simulink model "GCAWS"  (R2022a)
settings: Solver=FixedStepDiscrete  StartTime=0.0  StopTime=1  FixedStep=0.04  RelTol=1e-3
PreLoadFcn:
  | % Add Module Path
  | listing = dir;
  | if (contains([listing .name], 'TCAF')) && (contains([listing .name], 'MAP'))
  |     addpath('./TCAF', './MAP');
  |     addpath( genpath('./MAP') );
  | elseif (contains([listing .name], 'GCAWS.slx'))
  |     addpath('../TCAF', '../MAP');
  |     addpath( genpath('../MAP') );
  | else
  | end
  | 
  | % Add DataBus Path
  | load('BusStructureGCAWS.mat');
  | load('BusStructureWTPG.mat');
  | load('TRN\BusStructureTRN.mat');
InitFcn:
  | % Add Module Path
  | listing = dir;
  | if (contains([listing .name], 'TCAF')) && (contains([listing .name], 'MAP'))
  |     addpath('./TCAF', './MAP');
  |     addpath( genpath('./MAP') );
  | elseif (contains([listing .name], 'GCAWS.slx'))
  |     addpath('../TCAF', '../MAP');
  |     addpath( genpath('../MAP') );
  | else
  | end
  | 
  | % Add DataBus Path
  | load('BusStructureGCAWS.mat');
  | load('BusStructureWTPG.mat');
  | load('TRN\BusStructureTRN.mat');
StartFcn:
  | % Add Module Path
  | listing = dir;
  | if (contains([listing .name], 'TCAF')) && (contains([listing .name], 'MAP'))
  |     addpath('./TCAF', './MAP');
  |     addpath( genpath('./MAP') );
  | elseif (contains([listing .name], 'GCAWS.slx'))
  |     addpath('../TCAF', '../MAP');
  |     addpath( genpath('../MAP') );
  | else
  | end
  | 
  | % Add DataBus Path
  | load('BusStructureGCAWS.mat');
  | load('BusStructureWTPG.mat');
  | load('TRN\BusStructureTRN.mat');
values from neighbouring files (symbols this model uses):
  isFeasible = logsout{idx_WTPGDatapump}.Values.isFeasible.Data(ii,:)    [WTPG_SIM_AFTERPLOT.m]
undefined symbols (not defined in the file or in its folder): accNED, C_b_n, collisionWarning, collisionWarningValid, gOnsetRateWrap, lla, maxFlightPathAngleWrap, offObstructionMap, offTerrainMap, params, paramSelectedValid, pullUpGWrap, reactionTimeWrap, rollRateWrap, selectedWrap, statusCode, timeToGoToPullUp, velNED
libraries: hdlsllib x15, simulink x2
(part 2 of 2)

== matlab function GCAWS/ImplementGCAWS/CheckCollision/FindPullUpTimeLeft/BisectPullUpTimeBackup ==
  data: collisionFlag input; collisionIndex input; pullUpT output; predTraj input; hulledProfile input
function pullUpT = BisectPullUpTime(collisionFlag, collisionIndex, predTraj, hulledProfile)
%BisectPullUpTime
% == Output =======
% pullUpT : Time to pull-up time left [sec]

% Initailize output
pullUpT = single(10);
pullUpTD = 0;
terrHR = 0;
terrHL = 0;
terrTest = 0;

DELTA_T = 0.5;

% % If no collision found in the projected trajectory, return
% if collisionFlag(1) == 10
%     pullUpT = single(10);
%     return
% end

% If no collision found in pull-up trajectories, return
if (collisionFlag(2) == 65535) || (collisionFlag(1) == 65535) || (collisionIndex(2) == 65535)
    pullUpT = single(10);
    return
elseif ( (collisionIndex(2)-1) == 0 )
    % Collision now
    pullUpT = single(0);
    return;
else
    % Initialize TTGTPU
    pullUpTD = double( collisionIndex(2)-1 ) * DELTA_T;
    % Terrain Height at collision detected point
    terrHR = double( hulledProfile(collisionIndex(2)) );

    stateL = [ predTraj(collisionIndex(2)-1, collisionFlag(2), 1), ...
        predTraj(collisionIndex(2)-1, collisionFlag(2), 2), ...
        predTraj(collisionIndex(2)-1, collisionFlag(2), 3), ...
        pullUpTD-DELTA_T ];
    stateR = [ predTraj(collisionIndex(2), collisionFlag(2), 1), ...
        predTraj(collisionIndex(2), collisionFlag(2), 2), ...
        predTraj(collisionIndex(2), collisionFlag(2), 3), ...
        pullUpTD ];
    % Terrain height just before collision detected point
    terrHL = double( hulledProfile(collisionIndex(2)-1) );

    for bb = 0:12
        % Test terrain height

        terrTest = terrHL * ( (pullUpTD - (stateL(4) + stateR(4))/2 ) / DELTA_T) + ...
            terrHR * ( 1 - (pullUpTD - (stateL(4) + stateR(4))/2 ) / DELTA_T);

%         if ( abs(terrTest-((stateL(3) + stateR(3))/2)) < 0.01 )
%             break;
%         end

        if ( terrTest > ((stateL(3) + stateR(3))/2) )
            stateR(1) = (stateL(1) + stateR(1)) /2;
            stateR(2) = (stateL(2) + stateR(2)) /2;
            stateR(3) = (stateL(3) + stateR(3)) /2;
            stateR(4) = (stateL(4) + stateR(4)) /2;

        else
            stateL(1) = (stateL(1) + stateR(1)) /2;
            stateL(2) = (stateL(2) + stateR(2)) /2;
            stateL(3) = (stateL(3) + stateR(3)) /2;
            stateL(4) = (stateL(4) + stateR(4)) /2;

        end
    end

end

pullUpT = single( (stateL(4) + stateR(4))/2 );

end

== matlab function GCAWS/ImplementGCAWS/PredictTrajectory/GetProjectTrajectory ==
  data: GCAWSParam input; predTraj input; eulerDeg input; velXYZ input; velNED input; accXYZ input; lla input; predTraj output
function predTraj = GetProjectTrajectory(GCAWSParam, predTraj, eulerDeg, velXYZ, velNED, accXYZ, lla)
%GetProjectTrajectory GCAWS 명목 궤적 생성
%
% == Input =========
% GCAWSParam = [reactT; gMax; rollRate; gRate; gammaMax]
% predTraj - size of [41, 12, 3]
% eulerDeg = [roll; pitch; heading] (deg)
% velXYZ = [celX; velY; velZ] (mps)
% velNED = [velN; velE; velD] (mps)
% accXYZ = [accX; accY; accZ] (mps2)
% lla = [latitude_deg; longitude_deg; altitude_msl_m]
% DELTA_T = 0.5
% == Output ========
% predTraj = [41, 12, 3]
% 

% Define Constants
ALONG_TRACK_STEPS = size(predTraj, 1);
DELTA_T = 0.5;

%% Trajectory Prediction

% <1> Non-Pull-Up Scenario
predTraj(:, 1, :) = projectTrajcetory(eulerDeg, velXYZ, velNED, accXYZ, lla, ALONG_TRACK_STEPS, DELTA_T);
end

%% Internal functions
function nominal = projectTrajcetory(eulerDeg, velXYZ, velNED, accXYZ, lla, ALONG_TRACK_STEPS, DELTA_T)
%PROJECTTRAJECTORY
% Nominal Trajcetory 명목 궤적 예측
%       - Assumption 1: current aircraft sate is 100% reliable
%       - Assumption 2: aircraft maneuver is maintained

% Define constants
GRAV_ACC = 9.8;
LIMIT_TAN_ROL = 4;
LIMIT_TURN_RATE = 0.222; % [rad/s]
RAD2DEG = 180/pi;

assert (ALONG_TRACK_STEPS <= 81);

% Input Handling
rol = eulerDeg(1);
pit = eulerDeg(2);
hdg = eulerDeg(3);

velX = velXYZ(1);
velY = velXYZ(2);
velZ = velXYZ(3);

velN = velNED(1);
velE = velNED(2);
velD = velNED(3);

lat = lla(1);
lon = lla(2);
alt = lla(3);

% Flight path angle (deg)
gamma = atan2d(-velD, sqrt(velN^2+velE^2));

% Inertial speed
iSpd = sqrt( velX^2 + velY^2 + velZ^2 );
    
% Saturate inertial speed (since TAS is unavailable, use inertial spd) 
iSpd = saturate(iSpd, 0.1, 500);

% Calculate the length of a degree
[latLength, lonLength] = getLengthOfADegree(lat, alt);

velLat = velN / latLength;
velLon = velE / lonLength;

% Initialize Predicted Trajectory
nominal = zeros(ALONG_TRACK_STEPS, 1, 3);

% Start point
nominal(1, 1, 1) = lat;
nominal(1, 1, 2) = lon;
nominal(1, 1, 3) = alt;

for ii = 2:ALONG_TRACK_STEPS
    
    % [1] Update Attitude
    
    % Saturate tangent of roll (max bank angle = 75.9630 deg)
    tanRol = saturate(tand(rol), -LIMIT_TAN_ROL, LIMIT_TAN_ROL);
    
    % Saturate inertial speed (since TAS is unavailable, use inertial spd) 
    iSpd = saturate(iSpd, 0.1, 500);
    
    % Calculate turn rate [rad/s]
    turnRate = GRAV_ACC * tanRol / iSpd;
    
    % Saturate turn rate 
    turnRate = saturate(turnRate, -LIMIT_TURN_RATE, LIMIT_TURN_RATE);
        
    % Update heading [deg]
    hdg = hdg + turnRate * DELTA_T * RAD2DEG;
        
    % Update Flight Path Angle [deg]
    %        reaction time: 1.5 sec
    %        rate of change: 5 deg/s
    if ii < 4
        gamma = gamma;
    elseif gamma < -(5*DELTA_T)
        gamma = gamma + 5 * DELTA_T;
    elseif gamma < 0.0
        gamma = 0.0;
    else
        gamma = gamma;
    end

    % [2] Update Velocity
    velNTmp = sqrt(velN^2+velE^2+velD^2)*cosd(hdg)*cosd(gamma);
    velE    = sqrt(velN^2+velE^2+velD^2)*sind(hdg)*cosd(gamma);
    velN    = velNTmp;
    velDOld = velD;
    velD    = - sqrt(velN^2+velE^2+velD^2)*sind(gamma);

    % [3] Update Position
    % Rate of change in geodetic coordinates [deg/s]
    [latLength, lonLength] = getLengthOfADegree(nominal(ii, 1, 1), nominal(ii, 1, 3));
    velLatOld = velLat;
    velLonOld = velLon;
    velLat  = velN / latLength;
    velLon  = velE / lonLength;
    
    nominal(ii, 1, 1) = nominal(ii-1, 1, 1) + (velLat + velLatOld)/2 * DELTA_T;
    nominal(ii, 1, 2) = nominal(ii-1, 1, 2) + (velLon + velLonOld)/2 * DELTA_T;
    nominal(ii, 1, 3) = nominal(ii-1, 1, 3) - (velD + velDOld)/2 * DELTA_T;

end

end

function out = saturate(in, minVal, maxVal)
%SATURATE
% Saturates input value to [min, max]
%
% == Inputs =========
% in                - input value
% minVal            - minimum value
% maxVal            - maximum value
% == Outputs ========
% out               - saturated output value
% ===================

out = min(maxVal, max(minVal, in));

end

function [latLength, lonLength] = getLengthOfADegree(lat, h)
%GETLENGTHOFADEGREE
% Calculate the length of one degree of both latitude and longitude
% for a specified latitude and height
%
% == Inputs =========
% lat               - Latitude [deg]
% h                 - Height [m]
% 
% == Outputs ========
% latLength         - Length of 1 deg of latitude on the ref. spheroid [m]
% lonLength         - Length of 1 deg of longitude on the ref. spheroid [m]
% ===================

% WGS84 Parameters
eRadius = 6378137.0;
eEccen = 0.08181919;

% Radius of curvature in prime vertical
nE = eRadius / sqrt( 1 - (eEccen^2*(sind(lat))^2) );
% Meridian Radius of Curavature
mE = eRadius * (1 - eEccen^2) / (1 - eEccen^2*(sind(lat))^2)^(1.5);

lonLength = (nE + h) * cosd(lat) * (pi/180);
latLength = (mE + h) * (pi/180);

end

== matlab function GCAWS/HandleGCAWSInput/ConvertBody2NED ==
  data: eulerDeg input; vecNED output; vecXYZ input; C_b_n output
function [vecNED, C_b_n] = ConvertBody2NED(eulerDeg, vecXYZ)
%CONVERTBODY2NED 동체 좌표계 벡터를 NED 좌표계 벡터로 변환
% Body2NED 변환 행렬 출력

% Initialize
vecNED = zeros(3,1);
C_b_n = zeros(3,3);

% Trigonometirc functions
cRol = cosd(eulerDeg(1));
sRol = sind(eulerDeg(1));
cPit = cosd(eulerDeg(2));
sPit = sind(eulerDeg(2));
cYaw = cosd(eulerDeg(3));
sYaw = sind(eulerDeg(3));

% Transformation matrix
C_b_n   = [ cPit*cYaw, sRol*sPit*cYaw-cRol*sYaw, cRol*sPit*cYaw+sRol*sYaw;...
            cPit*sYaw, sRol*sPit*sYaw+cRol*cYaw, cRol*sPit*sYaw-sRol*cYaw;...
                -sPit,                sRol*cPit,                cRol*cPit];

% Transform
vecNED = C_b_n * vecXYZ;

end

== matlab function GCAWS/ImplementGCAWS/CheckCollision/FindCollisionFlag ==
  data: collision input; collisionFlag output; collisionIndex output
function [collisionFlag, collisionIndex] = FindCollisionFlag(collision)
%FINDCOLLISIONFLAG 지형충돌 플래그 생성
% == Output ===========
% collisionFlag
%  [1] = "collision", [65535] = "no collision"
% collisionIndex
%  [~] = "collision index", [65535] = "no collision"

% Initialize outputs
collisionFlag = uint16([65535 65535]);
collisionIndex= uint16([65535 65535]);

alongTrackSteps = size(collision, 1);

% <1> Already Below SWH
if any(collision(1:2,1), 'all')
    % Collision within 0.5 sec
    collisionFlag(1) = uint16(1);
    collisionIndex(1) = uint16(1);
else
    % Collision does not occur in 0.5 sec.
    collisionFlag(1) = uint16(65535);
    collisionIndex(1) = uint16(65535);
end

% <2> Pull-up Scenarios
% for ii = 1:41
%     % Collsiion at ii-th time index3
%     if any(collision(ii, 2:12), 'all')
%         collisionIndex(2) = uint16(ii);
%         % Find the fastest among collision case
%         collisionFlag(2) = uint16( 1 + find(collision(ii, 2:12), 1) );
% 
%         break
%     else
% 
%     end
% end

for jj = 2:12
    if any(collision(:, jj), 'all')
        % Collision at jj-th pull-up
        collisionFlag(2) = uint16(jj);
        collisionIndex(2) = find(collision(:, jj), 1);
        break
    end
end

% 
% for jj = 2:12
%     
%     if any(collision(1:41,jj), 'all')
%         % Collision at j-th pull-up
%         collisionFlag(2) = uint16(jj);
%         
%         % Find first collision
%         for ii = 1:alongTrackSteps
%             if collision(ii, jj)
%                 collisionIndex(2) = uint16(ii);
%                 break;
%             end
%         end
%         
%         break;
%     else
%         % Collision does not occur at j-th pull-up.
%         
%     end
%   
% end

end

== matlab function GCAWS/ImplementGCAWS/CheckCollision/FindPullUpTimeLeft/BisectPullUpTime ==
  data: collisionFlag input; collisionIndex input; pullUpT output; predTraj input; hulledProfile input; warning output; warningValid output
function [pullUpT, warning, warningValid]  = BisectPullUpTime(collisionFlag, collisionIndex, predTraj, hulledProfile)
%BisectPullUpTime
% == Output =======
% pullUpT : Time to pull-up time left [sec]
% warning
% warningValid

% Initailize output
pullUpT = single(5);
warning = false;
warningValid = true;

pullUpTD = 0;
terrHR = 0;
terrHL = 0;
terrTest = 0;

DELTA_T = 0.5;

% % If no collision found in the projected trajectory, return
% if collisionFlag(1) == 10
%     pullUpT = single(10);
%     return
% end

% If no collision found in pull-up trajectories, return
if (collisionFlag(2) == 65535) || (collisionIndex(2) == 65535)
    pullUpT = single(5);
    warning = false;
    warningValid = true;
    return
% Collision now
elseif ( collisionIndex(2) == 1 ) || ( collisionFlag(2) == 2) || (collisionFlag(1) == 1)
    pullUpT = single(0);
    warning = true;
    warningValid = true;
    return
else
    % Initialize TTGTPU
    pullUpTD = double( collisionFlag(2)-2 ) * DELTA_T;
    
    % Terrain Height at collision detected point
    terrHR = double( hulledProfile(collisionIndex(2)) );
    terrTest = double( hulledProfile(collisionIndex(2)) );
    
    stateL = [ predTraj(collisionIndex(2), collisionFlag(2)-1, 1), ...
        predTraj(collisionIndex(2), collisionFlag(2)-1, 2), ...
        predTraj(collisionIndex(2), collisionFlag(2)-1, 3), ...
        pullUpTD-DELTA_T ];
    stateR = [ predTraj(collisionIndex(2), collisionFlag(2), 1), ...
        predTraj(collisionIndex(2), collisionFlag(2), 2), ...
        predTraj(collisionIndex(2), collisionFlag(2), 3), ...
        pullUpTD ];

    % Terrain height just before collision detected point
    terrHL = double( hulledProfile(collisionIndex(2)-1) );

    for bb = 0:12
        % Test terrain height
        terrTest = double( hulledProfile(collisionIndex(2)) );
%         terrTest = terrHL * ( (pullUpTD - (stateL(4) + stateR(4))/2 ) / DELTA_T) + ...
%             terrHR * ( 1 - (pullUpTD - (stateL(4) + stateR(4))/2 ) / DELTA_T);

        if ( terrTest > ((stateL(3) + stateR(3))/2) )
            stateR(1) = (stateL(1) + stateR(1)) /2;
            stateR(2) = (stateL(2) + stateR(2)) /2;
            stateR(3) = (stateL(3) + stateR(3)) /2;
            stateR(4) = (stateL(4) + stateR(4)) /2;

        else
            stateL(1) = (stateL(1) + stateR(1)) /2;
            stateL(2) = (stateL(2) + stateR(2)) /2;
            stateL(3) = (stateL(3) + stateR(3)) /2;
            stateL(4) = (stateL(4) + stateR(4)) /2;

        end
    end

end

pullUpT = single( (stateL(4) + stateR(4))/2 );

if (pullUpT > 0) && (pullUpT <= 5)
    warning = false;
    warningValid = true;
else
    warning = false;
    warningValid = false;
end

== matlab function GCAWS/ImplementGCAWS/CheckCollision/CheckProfileCollision ==
  data: hulledProfile input; collision output; predTraj input
function collision = CheckProfileCollision(hulledProfile, predTraj)
% CheckProfileCollision 프로파일별 지형 충돌여부 검사
%
% == Output ============
% collision : [41, 12]
%             tIdx, # of profile

%
collision = zeros(41, 12, 'logical');
alongTrackSteps = size(hulledProfile, 1);

% Check Collision
for jj = 1:12
    
    for ii = 1:alongTrackSteps
        
        collision(ii, jj) = (predTraj(ii, jj, 3) <= hulledProfile(ii));
        
    end
    
end

== matlab function GCAWS/ImplementGCAWS/HullProfile/GetHulledProfile ==
  data: wtp input; hulled output; swh input; gcawsParams input; speed input; VerticalUncertainty input
function hulled = GetHulledProfile(wtp, swh, gcawsParams, speed, VerticalUncertainty)
%GETHULLEDPROFILE 헐링 프로파일을 생성
assert ( all ( size (wtp) == [41 1 ] ) )
assert ( isscalar(swh) )
assert ( all ( size (gcawsParams) == [5 1 ] ) )
assert ( isscalar(speed) )
assert ( isscalar(VerticalUncertainty) )

% Profile Hulling Activation Flag
IS_HULLED = false; % Hulling is deactivated in order not to interfere
% MATLAB Script Debugging Flag
ON_DEBUG = false;

% -- START: ON_DEBUG ------------------------------------------------------
% if ON_DEBUG
%     wtp = ones( 41, 1, 'single') * 100;
%     for ii = 2:41
%         if abs(randn) < 0.2 
%             wtp(ii) = wtp(ii-1);
%         else
%             wtp(ii) = single( wtp(ii-1) + ceil(randn * 10) );
%         end
%     end
%     swh = 30.48;
%     params = [1.5, 120, 4.0, 4.0, 75];
%     % (1) Reaction Time (sec)
%     % (2) Max Pull Up G (g)
%     % (3) Roll Rate (deg/s)
%     % (4) G Onset Rate (g/s)
%     % (5) Max Flight Path Angle (deg)
%     VerticalUncertainty = 20;
%     wtpTime = 0:0.5:20;
% end
% -- END: ON_DEBUG --------------------------------------------------------

% Length of Worst-case Terrain Profile
wtpLength = size(wtp, 1);

% Initialize
hulled = zeros(wtpLength, 1, 'single');
hullIdx = zeros(wtpLength, 1, 'uint8');
hulltemp = wtp;

a = gcawsParams(2) * 9.81;
theta = gcawsParams(5) * (pi/180);
v = speed;

% If Hulling Activated
if IS_HULLED
    
    % Sort profile in descending order
    [~, hullIdx] = sort(wtp, 'descend');

    for kk = 2:length(hullIdx)
        changed = false;

        for ii = 2:length(hullIdx)
            % ※제일 높은 1번째 인덱스는 검사할 필요 없음

            % I번째 검사지점
            curI = hullIdx(ii);
            dh = single(0.0);

            % I번째보다 높은 (I-1)부터 1까지 비교하였을 때
            for jj = (ii-1):-1:1
                curJ = hullIdx(jj);
                dt = (curJ - curI) * 0.5;

                if hulltemp(curJ) > ( hulltemp(curI) + GetProbeHeight(a, theta, v, dt))

                    dhTemp = ( hulltemp(curJ) - ( hulltemp(curI) + GetProbeHeight(a, theta, v, dt)) );
                    if dhTemp > dh
                        dh =dhTemp;
                    else
                    end
                else
                end

            end
            if dh > 0
                hulltemp(curI) = hulltemp(curI) + dh;
                changed = true;
            else
            end

        end

        % Terimination Condition
        if changed
            % If changed, sort profile and do hulling again.
            [~, hullIdx] = sort(hulltemp, 'descend');
            continue
        else
            break
        end

    end

end

% Output
hulled = hulltemp + swh + 2 * VerticalUncertainty;

% -- START: ON_DEBUG ------------------------------------------------------
% if ON_DEBUG
%     figure('WindowStyle', 'docked')
%     hold on;
%     plot(wtpTime, wtp, '.-b', 'DisplayName', 'Worst-case Terrain Profile');
%     plot(wtpTime, hulltemp, '-r', 'DisplayName', 'Hulled Profile');
% 
%     time = -1.5:0.5:1.5;
% 
%     for ii = 1:length(hulltemp)
%         y = zeros(size(time));
%         t = time + (ii-1)*0.5;
%         for jj = 1:length(time)
%             y(jj) = hulltemp(ii) + GetProbeHeight(a, theta, v, time(jj));
%         end
%         if ii == 1
%             plot(t, y, ':', 'Color', [0.4 0.4 0.4], 'DisplayName', 'Probe profile');
%         else
%             plot(t, y, ':', 'Color', [0.4 0.4 0.4], 'HandleVisibility', 'off');
%         end
% 
%     end
%     % plot(wtpTime, hulled, '-m', 'DisplayName', 'Hulled + SWH + Uncertainty Profile');
%     legend('Location', 'best');
%     hold off;
%     grid minor
%     xlabel('Time (sec)');
%     ylabel('Height (m)');
% end
% -- END: ON_DEBUG --------------------------------------------------------

end

%% subfunctions
function y = GetProbeHeight(a, theta, v, t)

R = v^2 / a;
w = a / v;
T = theta / w;

if (abs(t) > T)
    y = single( R - R*cos(theta) + v*sin(theta)*( abs(t) -abs(T) ) );
else
    y = single( R - R*cos(w*t) );
end

end

== matlab function GCAWS/ImplementGCAWS/PredictTrajectory/predictTrajectoryGCAWS ==
  data: GCAWSParam input; predTraj input; eulerDeg input; velXYZ input; velNED input; accXYZ input; lla input; predTraj output; DELTA_T input
function predTraj = predictTrajectoryGCAWS(GCAWSParam, predTraj, eulerDeg, velXYZ, velNED, accXYZ, lla, DELTA_T)
%PREDICTTRAJECTORYGCAWS GCAWS 기준/회복궤적 생성
%
% == Input =========
% GCAWSParam = [reactT; gMax; rollRate; gRate; gammaMax]
% predTraj - size of [41, 12, 3]
% eulerDeg = [roll; pitch; heading] (deg)
% velXYZ = [celX; velY; velZ] (mps)
% velNED = [velN; velE; velD] (mps)
% accXYZ = [accX; accY; accZ] (mps2)
% lla = [latitude_deg; longitude_deg; altitude_msl_m]
% DELTA_T = 0.5
% == Output ========
% predTraj = [41, 12, 3]
% 

% Define Constants
GRAV_ACC = 9.8;
ALONG_TRACK_STEPS = size(predTraj, 1);

%% Trajectory Prediction

% <1> Non-Pull-Up Scenario
predTraj(:, 1, :) = projectTrajcetory(eulerDeg, velXYZ, velNED, accXYZ, lla, ALONG_TRACK_STEPS, DELTA_T);

% <2> Pull-Up Scenario
for jj = 2:12
    % [jj=2: 바로 Pull-up 기동; jj=3: 0.5초 후 Pull-up 기동; ... ; jj=k: (k-2)*0.5초 후 Pull-up 기동] 
    predTraj(:, jj, :) = pullUpTrajectory(GCAWSParam, eulerDeg, velXYZ, velNED, accXYZ, lla, ALONG_TRACK_STEPS, DELTA_T, jj-2);
end

end
%% sub-functions
function pullUp = pullUpTrajectory(gcawsParam, eulerDeg, velXYZ, velNED, accXYZ, lla, ALONG_TRACK_STEPS, DELTA_T, pullUpTIdx)
%PULLUPTRAJECTORY
% Pull-up Trajectry 풀업 비행경로 예측

% Define constants
GRAV_ACC = 9.8;
RAD2DEG = 180/pi;
LIMIT_TAN_ROL = 4;
LIMIT_TURN_RATE = 0.222; % [rad/s]

assert (ALONG_TRACK_STEPS <= 81);

% Input Handling
rol = eulerDeg(1);
pit = eulerDeg(2);
hdg = eulerDeg(3);

velX = velXYZ(1);
velY = velXYZ(2);
velZ = velXYZ(3);

velN = velNED(1);
velE = velNED(2);
velD = velNED(3);

accNED = zeros(3,1);

lat = lla(1);
lon = lla(2);
alt = lla(3);

reactT = gcawsParam(1);     % [sec]
if velD > 0
    % 항공기 하강 시에Reaction Time을 0.5초 * Sin(비행경로 각도)만큼 증가
    gamma = atan2(velD, sqrt(velN^2 + velE^2));
    reactT = gcawsParam(1) + 0.5 * sin(gamma);
else
    reactT = gcawsParam(1); % [sec]
end

upGMax = gcawsParam(2);     % [g]
rollRate = gcawsParam(3);   % [deg/s]
gRate = gcawsParam(4);      % [g/s]
gammaMax = gcawsParam(5);   % [deg]

% Inertial speed
iSpd = sqrt( velX^2 + velY^2 + velZ^2 );
    
% Saturate inertial speed (since TAS is unavailable, use inertial spd) 
iSpd = saturate(iSpd, 0.1, 500);

% Calculate the length of a degree
[latLength, lonLength] = getLengthOfADegree(lat, alt);

velLat = velN / latLength;
velLon = velE / lonLength;

% Initialize Predicted Trajectory
pullUp = zeros(ALONG_TRACK_STEPS, 1, 3);
pullUp(1, 1, :) = lla;

% Time slices
% - Pull-up Timing (t1Idx = 1)
t1Idx = 1 + pullUpTIdx;
% - Reaction Tiem (t2Idx = 4.2)
t2Idx = t1Idx + (reactT/DELTA_T);
% - Roll Recovery (t3Idx = 4.3667)
t3Idx = t2Idx + abs( rol/rollRate )/DELTA_T;

for ii = 2:ALONG_TRACK_STEPS
    
    if ii <= t2Idx
        % [1] Projected & Pilot Reaction 
        % [1.1] Update Attitude

        % Saturate tangent of roll (max bank angle = 75.9630 deg)
        tanRol = saturate(tand(rol), -LIMIT_TAN_ROL, LIMIT_TAN_ROL);

        % Saturate inertial speed (since TAS is unavailable, use inertial spd)
        iSpd = saturate(iSpd, 0.1, 500);

        % Calculate turn rate [rad/s]
        turnRate = GRAV_ACC * tanRol / iSpd;

        % Saturate turn rate
        turnRate = saturate(turnRate, -LIMIT_TURN_RATE, LIMIT_TURN_RATE);

        % Update heading [deg]
        hdg = hdg + turnRate * DELTA_T * RAD2DEG;

        % [1.2] Update Velocity
        velNTmp = sqrt(velN^2+velE^2)*cosd(hdg);
        velE    = sqrt(velN^2+velE^2)*sind(hdg);
        velN    = velNTmp;
        velDOld = velD;

        if ii == 2
            % Update Velocity with Acceleration only when first time
            % Body2NED to get accNED
            [accNED, ~] = convertBody2NED(eulerDeg, accXYZ);
            
            % Update velocity (Acceleration is assumed to be diminishing)
            velN = velN + (accNED(1) + 0)/2 * DELTA_T;
            velE = velE + (accNED(2) + 0)/2 * DELTA_T;
            velD = velD + (accNED(3) + 0)/2 * DELTA_T;
        end

        % [1.3] Update Position
        % Rate of change in geodetic coordinates [deg/s]
        if mod(ii, 41) == 0
            [latLength, lonLength] = getLengthOfADegree(pullUp(ii, 1, 1), pullUp(ii, 1, 3));
        end
        velLatOld = velLat;
        velLonOld = velLon;
        velLat  = velN / latLength;
        velLon  = velE / lonLength;
        
        pullUp(ii, 1, 1) = pullUp(ii-1, 1, 1) + (velLat + velLatOld)/2 * DELTA_T;
        pullUp(ii, 1, 2) = pullUp(ii-1, 1, 2) + (velLon + velLonOld)/2 * DELTA_T;
        pullUp(ii, 1, 3) = pullUp(ii-1, 1, 3) - (velD + velDOld)/2 * DELTA_T;
        
    elseif (ii > t2Idx) && ( ii <= t3Idx )
        % [2] Roll recovery
        if ii == ceil(t2Idx)
            DELTA_T_rolRec = DELTA_T * (ii - t2Idx);
        else
            DELTA_T_rolRec = DELTA_T;
        end

        % [2.1] Update Attitude
        rolOld = rol;
        rol = rol - sign(rol) * rollRate * DELTA_T_rolRec;
        
        if sign(rol) ~= sign(rolOld) 
            rol = 0;
        end
        
        % Saturate tangent of roll (max bank angle = 75.9630 deg)
        tanRol = saturate(tand(rol), -LIMIT_TAN_ROL, LIMIT_TAN_ROL);
        tanRolOld = saturate(tand(rolOld), -LIMIT_TAN_ROL, LIMIT_TAN_ROL);

        % Saturate inertial speed (since TAS is unavailable, use inertial spd) 
        iSpd = saturate(iSpd, 0.1, 500);
        
        % Calculate turn rate [rad/s]
        turnRate = GRAV_ACC * tanRol / iSpd;
        turnRateOld = GRAV_ACC * tanRolOld / iSpd;

        % Saturate turn rate 
        turnRate = saturate(turnRate, -LIMIT_TURN_RATE, LIMIT_TURN_RATE);
        turnRateOld = saturate(turnRateOld, -LIMIT_TURN_RATE, LIMIT_TURN_RATE);
        
        % Update heading [deg]
        hdg = hdg + (turnRate + turnRateOld)/2 * DELTA_T_rolRec * RAD2DEG;
        
        % [2.2] Update Velocity
        velNTmp = sqrt(velN^2+velE^2)*cosd(hdg);
        velE    = sqrt(velN^2+velE^2)*sind(hdg);
        velN    = velNTmp;
        velDOld = velD;
        
        u = sqrt(velN^2 + velE^2);
        pit = -velD/u * RAD2DEG;
        
        % [2.3] Update Position
        % Rate of change in geodetic coordinates [deg/s]
        if mod(ii, 41) == 0
            [latLength, lonLength] = getLengthOfADegree(pullUp(ii, 1, 1), pullUp(ii, 1, 3));
        end
        velLatOld = velLat;
        velLonOld = velLon;
        velLat  = velN / latLength;
        velLon  = velE / lonLength;
        
        pullUp(ii, 1, 1) = pullUp(ii-1, 1, 1) + (velLat + velLatOld)/2 * DELTA_T;
        pullUp(ii, 1, 2) = pullUp(ii-1, 1, 2) + (velLon + velLonOld)/2 * DELTA_T;
        pullUp(ii, 1, 3) = pullUp(ii-1, 1, 3) - (velD + velDOld)/2 * DELTA_T;

    elseif ii > t3Idx
        % [3&4] Pull-up Maneuver
        rolOld = rol;
        rol = 0;
        
        if ii == ceil(t3Idx)
            DELTA_T_pullUp = DELTA_T * (ii - t3Idx);
        else
            DELTA_T_pullUp = DELTA_T;
        end

        
        gNED = [0; 0; GRAV_ACC];
        [~, C_b_n] = convertBody2NED(eulerDeg, [1; 1; 1]);
        C_n_b = C_b_n';
        
        gXYZ = C_n_b * gNED;
        
        if abs( GRAV_ACC/cosd(pit) ) > upGMax * GRAV_ACC
            accXYZ	=  [0; 0; -upGMax*GRAV_ACC] + gXYZ;
        else
            accXYZ = [0; 0; -abs( GRAV_ACC/cosd(pit) )] + gXYZ;
        end
        
        az = accXYZ(3);
        pit = pit - ( (az + GRAV_ACC*cosd(pit) ) / velX) * RAD2DEG * DELTA_T_pullUp;
        
        velDOld = velD;
        if abs(pit) < gammaMax
        % third step - g on set rate with pull up G
            
            az = az - gRate*GRAV_ACC*DELTA_T_pullUp;
            az = saturate(az, -upGMax*GRAV_ACC, upGMax*GRAV_ACC);
            aTmp = [0, 0, az]';
            [accNED, ~] = convertBody2NED([rol, pit, hdg], aTmp);

            velN = velN + accNED(1)*DELTA_T_pullUp;
            velE = velE + accNED(2)*DELTA_T_pullUp;
            velD = velD + accNED(3)*DELTA_T_pullUp;
        
        else
        % fourth step - Maximum flight path angle rising
            pit = sign(pit) * gammaMax;
        end
        
        % [3.3] Update Position
        % Rate of change in geodetic coordinates [deg/s]
        if mod(ii, 41) == 0
            [latLength, lonLength] = getLengthOfADegree(pullUp(ii, 1, 1), pullUp(ii, 1, 3));
        end
        velLatOld = velLat;
        velLonOld = velLon;
        velLat  = velN / latLength;
        velLon  = velE / lonLength;
        
        pullUp(ii, 1, 1) = pullUp(ii-1, 1, 1) + (velLat + velLatOld)/2 * DELTA_T;
        pullUp(ii, 1, 2) = pullUp(ii-1, 1, 2) + (velLon + velLonOld)/2 * DELTA_T;
        pullUp(ii, 1, 3) = pullUp(ii-1, 1, 3) - (velD + velDOld)/2 * DELTA_T;
        
    end
    
end

end


function nominal = projectTrajcetory(eulerDeg, velXYZ, velNED, accXYZ, lla, ALONG_TRACK_STEPS, DELTA_T)
%PROJECTTRAJECTORY
% Nominal Trajcetory 명목 궤적 예측
%       - Assumption 1: current aircraft sate is 100% reliable
%       - Assumption 2: aircraft maneuver is maintained

% Define constants
GRAV_ACC = 9.8;
LIMIT_TAN_ROL = 4;
LIMIT_TURN_RATE = 0.222; % [rad/s]
RAD2DEG = 180/pi;

assert (ALONG_TRACK_STEPS <= 81);

% Input Handling
rol = eulerDeg(1);
pit = eulerDeg(2);
hdg = eulerDeg(3);

velX = velXYZ(1);
velY = velXYZ(2);
velZ = velXYZ(3);

velN = velNED(1);
velE = velNED(2);
velD = velNED(3);

lat = lla(1);
lon = lla(2);
alt = lla(3);

% Inertial speed
iSpd = sqrt( velX^2 + velY^2 + velZ^2 );
    
% Saturate inertial speed (since TAS is unavailable, use inertial spd) 
iSpd = saturate(iSpd, 0.1, 500);

% Calculate the length of a degree
[latLength, lonLength] = getLengthOfADegree(lat, alt);

velLat = velN / latLength;
velLon = velE / lonLength;

% Initialize Predicted Trajectory
nominal = zeros(ALONG_TRACK_STEPS, 1, 3);

% Start point
nominal(1, 1, 1) = lat;
nominal(1, 1, 2) = lon;
nominal(1, 1, 3) = alt;

for ii = 2:ALONG_TRACK_STEPS
    
    % [1] Update Attitude
    
    % Saturate tangent of roll (max bank angle = 75.9630 deg)
    tanRol = saturate(tand(rol), -LIMIT_TAN_ROL, LIMIT_TAN_ROL);
    
    % Saturate inertial speed (since TAS is unavailable, use inertial spd) 
    iSpd = saturate(iSpd, 0.1, 500);
    
    % Calculate turn rate [rad/s]
    turnRate = GRAV_ACC * tanRol / iSpd;
    
    % Saturate turn rate 
    turnRate = saturate(turnRate, -LIMIT_TURN_RATE, LIMIT_TURN_RATE);
        
    % Update heading [deg]
    hdg = hdg + turnRate * DELTA_T * RAD2DEG;
        
    % [2] Update Velocity
    velNTmp = sqrt(velN^2+velE^2)*cosd(hdg);
    velE    = sqrt(velN^2+velE^2)*sind(hdg);
    velN    = velNTmp;
    velDOld = velD;

    % [3] Update Position
    % Rate of change in geodetic coordinates [deg/s]
    if mod(ii, 41) == 0
        [latLength, lonLength] = getLengthOfADegree(nominal(ii, 1, 1), nominal(ii, 1, 3));
    end
    velLatOld = velLat;
    velLonOld = velLon;
    velLat  = velN / latLength;
    velLon  = velE / lonLength;
    
    nominal(ii, 1, 1) = nominal(ii-1, 1, 1) + (velLat + velLatOld)/2 * DELTA_T;
    nominal(ii, 1, 2) = nominal(ii-1, 1, 2) + (velLon + velLonOld)/2 * DELTA_T;
    nominal(ii, 1, 3) = nominal(ii-1, 1, 3) - (velD + velDOld)/2 * DELTA_T;

end

end

function out = saturate(in, minVal, maxVal)
%SATURATE
% Saturates input value to [min, max]
%
% == Inputs =========
% in                - input value
% minVal            - minimum value
% maxVal            - maximum value
% == Outputs ========
% out               - saturated output value
% ===================

out = min(maxVal, max(minVal, in));

end

function [latLength, lonLength] = getLengthOfADegree(lat, h)
%GETLENGTHOFADEGREE
% Calculate the length of one degree of both latitude and longitude
% for a specified latitude and height
%
% == Inputs =========
% lat               - Latitude [deg]
% h                 - Height [m]
% 
% == Outputs ========
% latLength         - Length of 1 deg of latitude on the ref. spheroid [m]
% lonLength         - Length of 1 deg of longitude on the ref. spheroid [m]
% ===================

% WGS84 Parameters
eRadius = 6378137.0;
eEccen = 0.08181919;

% Radius of curvature in prime vertical
nE = eRadius / sqrt( 1 - (eEccen^2*(sind(lat))^2) );
% Meridian Radius of Curavature
mE = eRadius * (1 - eEccen^2) / (1 - eEccen^2*(sind(lat))^2)^(1.5);

lonLength = (nE + h) * cosd(lat) * (pi/180);
latLength = (mE + h) * (pi/180);

end

function [vecNED, C_b_n] = convertBody2NED(eulerDeg, vecXYZ)
%CONVERTBODY2NED 동체 좌표계 벡터를 NED 좌표계 벡터로 변환
% Body2NED 변환 행렬 출력

% Initialize
vecNED = zeros(3,1);
C_n_b = zeros(3,3);
C_b_n = zeros(3,3);

% Trigonometirc functions
cRol = cosd(eulerDeg(1));
sRol = sind(eulerDeg(1));
cPit = cosd(eulerDeg(2));
sPit = sind(eulerDeg(2));
cYaw = cosd(eulerDeg(3));
sYaw = sind(eulerDeg(3));

% Transformation matrix
C_n_b   = [              cPit*cYaw,                cPit*sYaw,     -sPit;...
          sRol*sPit*cYaw-cRol*sYaw, sRol*sPit*sYaw+cRol*cYaw, sRol*cPit;...
          cRol*sPit*cYaw+sRol*sYaw, cRol*sPit*sYaw-sRol*cYaw, cRol*cPit];

C_b_n   = C_n_b';

% Transform
if size(vecXYZ, 1) == 3
    vecNED = C_b_n * vecXYZ;
elseif size(vecXYZ, 2) == 3
    vecNED = C_b_n * vecXYZ';
else
    vecNED = [0; 0; 0];
    warning('Invalid input vectors for <convertBody2NED>');
end

end

== matlab function GCAWS/ImplementGCAWS/PredictTrajectory/PredictRecoveryTrajectory/GetRecoveryTrajectory ==
  data: gcawsParam input; pullUpTraj output; eulerDeg input; velXYZ input; velNED input; accXYZ input; lla input; recoveryTime input
function pullUpTraj = GetRecoveryTrajectory(gcawsParam, eulerDeg, velXYZ, velNED, accXYZ, lla, recoveryTime)
%GetRecoveryTrajectory
% == Input =========
% gcawsParam = [reactT; gMax; rollRate; gRate; gammaMax]
% eulerDeg = [roll; pitch; heading] (deg)
% velXYZ = [celX; velY; velZ] (mps)
% velNED = [velN; velE; velD] (mps)
% accXYZ = [accX; accY; accZ] (mps2)
% lla = [latitude_deg; longitude_deg; altitude_msl_m]
% == Output ========
% predTraj = [41, 12, 3]
% 

% Initialize Outputs
pullUpTraj = zeros(41, 1, 3);

% Define constants
DELTA_T = 0.5;
GRAV_ACC = 9.8;
RAD2DEG = 180/pi;
LIMIT_TAN_ROL = 4;
LIMIT_TURN_RATE = 0.222; % [rad/s]
ALONG_TRACK_STEPS = 41;
EPSILON = 0.00001;

% Input Handling
rol = eulerDeg(1);
pit = eulerDeg(2);
hdg = eulerDeg(3);

velX = velXYZ(1);
velY = velXYZ(2);
velZ = velXYZ(3);

velN = velNED(1);
velE = velNED(2);
velD = velNED(3);

accNED = zeros(3,1);

lat = lla(1);
lon = lla(2);
alt = lla(3);

% Flight path angle (deg)
gamma = atan2d(-velD, sqrt(velN^2+velE^2));


reactT = gcawsParam(1);     % [sec]

if velD > 0
    % 항공기 하강 시에 Reaction Time을 0.5초 * Sin(비행경로 각도)만큼 증가
    reactT = gcawsParam(1) + 0.5 * sind(gamma);

    % 항공기 하강 시에 현재 고도를 0.5초 * sin(비행경로각)만큼 더 하강한 것으로 가정
else
    reactT = gcawsParam(1); % [sec]
end

upGMax = gcawsParam(2);     % [g]
rollRate = gcawsParam(3);   % [deg/s]
gRate = gcawsParam(4);      % [g/s]
gammaMax = gcawsParam(5);   % [deg]

% Inertial speed
iSpd = sqrt( velX^2 + velY^2 + velZ^2 );

% Saturate inertial speed (since TAS is unavailable, use inertial spd)
iSpd = saturate(iSpd, 75.1089, 500);

% Calculate the length of a degree
[latLength, lonLength] = getLengthOfADegree(lat, alt);

velLat = velN / latLength;
velLon = velE / lonLength;

% Initial position
pullUpTraj(1, 1, :) = lla;

% Time slices
% - Pull-up Timing (t1Idx = 1)
t1Idx = 1 + (recoveryTime/DELTA_T);
% - Reaction Tiem (t2Idx = 4.2)
t2Idx = t1Idx + (reactT/DELTA_T);

% - Roll Recovery (t3Idx = 4.3667)
t3Idx = t2Idx + abs( rol/rollRate )/DELTA_T;

% fprintf("t2Idx: %.0f, t3Idx: %.0f \r\n", t2Idx, t3Idx);
[latLength, lonLength] = getLengthOfADegree(pullUpTraj(1, 1, 1), pullUpTraj(1, 1, 3));

for ii = 2:ALONG_TRACK_STEPS

    % Flight path angle (deg)
    gamma = atan2d(-velD, sqrt(velN^2+velE^2));

    %     % Update Flight Path Angle [deg]
    %     %        reaction time: 0.5 sec
    %     %        rate of change: 5 deg/s
    %     if ii < 2
    %         gamma = gamma;
    %     elseif gamma < -(10*DELTA_T)
    %         gamma = gamma + 5 * DELTA_T;
    %     elseif gamma < 0.0
    % %         gamma = 0.0;
    %         gamma = gamma + 5 * DELTA_T;
    %     else
    %         gamma = gamma;
    %     end
    gNED = [0; 0; GRAV_ACC];
    [~, C_b_n] = convertBody2NED(eulerDeg, [1; 1; 1]);
    C_n_b = C_b_n';

    gXYZ = C_n_b * gNED;

    if abs( GRAV_ACC/cosd(pit) ) > upGMax * GRAV_ACC
        accXYZ	=  [0; 0; -upGMax*GRAV_ACC] + gXYZ;
    else
        accXYZ = [0; 0; -abs( GRAV_ACC/cosd(pit) )] + gXYZ;
    end

    az = accXYZ(3);

    if ii <= t2Idx
        % [1] Projected & Pilot Reaction
        % [1.1] Update Attitude

        % Saturate tangent of roll (max bank angle = 75.9630 deg)
        tanRol = saturate(tand(rol), -LIMIT_TAN_ROL, LIMIT_TAN_ROL);

        % Saturate inertial speed (since TAS is unavailable, use inertial spd)
        iSpd = saturate(iSpd, 0.1, 500);

        % Calculate turn rate [rad/s]
        turnRate = GRAV_ACC * tanRol / iSpd;

        % Saturate turn rate
        turnRate = saturate(turnRate, -LIMIT_TURN_RATE, LIMIT_TURN_RATE);

        % Update heading [deg]
        hdg = hdg + turnRate * DELTA_T * RAD2DEG;

        % [2] Update Velocity
        velNTmp = sqrt(velN^2+velE^2+velD^2)*cosd(hdg)*cosd(gamma);
        velE    = sqrt(velN^2+velE^2+velD^2)*sind(hdg)*cosd(gamma);
        velN    = velNTmp;
        velDOld = velD;
        velD    = - sqrt(velN^2+velE^2+velD^2)*sind(gamma);

        if ii == 2
            % Update Velocity with Acceleration only when first time
            % Body2NED to get accNED
            [accNED, ~] = convertBody2NED(eulerDeg, accXYZ);

            % Update velocity (Acceleration is assumed to be diminishing)
            velN = velN + (accNED(1) + 0)/2 * DELTA_T;
            velE = velE + (accNED(2) + 0)/2 * DELTA_T;
            velD = velD + (accNED(3) + 0)/2 * DELTA_T;
        end

        % [1.3] Update Position
        % Rate of change in geodetic coordinates [deg/s]
        velLatOld = velLat;
        velLonOld = velLon;
        velLat  = velN / latLength;
        velLon  = velE / lonLength;

        pullUpTraj(ii, 1, 1) = pullUpTraj(ii-1, 1, 1) + (velLat + velLatOld)/2 * DELTA_T;
        pullUpTraj(ii, 1, 2) = pullUpTraj(ii-1, 1, 2) + (velLon + velLonOld)/2 * DELTA_T;
        pullUpTraj(ii, 1, 3) = pullUpTraj(ii-1, 1, 3) - (velD + velDOld)/2 * DELTA_T;

    elseif (ii > t2Idx) && ( ii <= t3Idx )
        % [2] Roll recovery
%         if ii == ceil(t2Idx)
        if abs(ii-ceil(t2Idx)) < EPSILON
            DELTA_T_rolRec = DELTA_T * (ii - t2Idx);
        else
            DELTA_T_rolRec = DELTA_T;
        end

        % [2.1] Update Attitude
        rolOld = rol;
        rol = rol - sign(rol) * rollRate * DELTA_T_rolRec;

        if (sign(rol*rolOld) < 0)
            rol = 0;
        end

        % Saturate tangent of roll (max bank angle = 75.9630 deg)
        tanRol = saturate(tand(rol), -LIMIT_TAN_ROL, LIMIT_TAN_ROL);
        tanRolOld = saturate(tand(rolOld), -LIMIT_TAN_ROL, LIMIT_TAN_ROL);

        % Saturate inertial speed (since TAS is unavailable, use inertial spd)
        iSpd = saturate(iSpd, 0.1, 500);

        % Calculate turn rate [rad/s]
        turnRate = GRAV_ACC * tanRol / iSpd;
        turnRateOld = GRAV_ACC * tanRolOld / iSpd;

        % Saturate turn rate
        turnRate = saturate(turnRate, -LIMIT_TURN_RATE, LIMIT_TURN_RATE);
        turnRateOld = saturate(turnRateOld, -LIMIT_TURN_RATE, LIMIT_TURN_RATE);

        % Update heading [deg]
        hdg = hdg + (turnRate + turnRateOld)/2 * DELTA_T_rolRec * RAD2DEG;

        % [2] Update Velocity
        velNTmp = sqrt(velN^2+velE^2+velD^2)*cosd(hdg)*cosd(gamma);
        velE    = sqrt(velN^2+velE^2+velD^2)*sind(hdg)*cosd(gamma);
        velN    = velNTmp;
        velDOld = velD;
        velD    = - sqrt(velN^2+velE^2+velD^2)*sind(gamma);

        u = sqrt(velN^2 + velE^2);
        pit = -velD/u * RAD2DEG;

        % [2.3] Update Position
        % Rate of change in geodetic coordinates [deg/s]
        velLatOld = velLat;
        velLonOld = velLon;
        velLat  = velN / latLength;
        velLon  = velE / lonLength;

        pullUpTraj(ii, 1, 1) = pullUpTraj(ii-1, 1, 1) + (velLat + velLatOld)/2 * DELTA_T;
        pullUpTraj(ii, 1, 2) = pullUpTraj(ii-1, 1, 2) + (velLon + velLonOld)/2 * DELTA_T;
        pullUpTraj(ii, 1, 3) = pullUpTraj(ii-1, 1, 3) - (velD + velDOld)/2 * DELTA_T;

    elseif ii > t3Idx
        % [3&4] Pull-up Maneuver
        rolOld = rol;
        rol = 0;

%         if ii == ceil(t3Idx)
        if abs(ii-ceil(t3Idx)) < EPSILON
            DELTA_T_pullUp = DELTA_T * (ii - t3Idx);
        else
            DELTA_T_pullUp = DELTA_T;
        end

        gNED = [0; 0; GRAV_ACC];
        [~, C_b_n] = convertBody2NED([rol; pit; hdg], [1; 1; 1]);
        C_n_b = C_b_n';

        gXYZ = C_n_b * gNED;

        pit = pit - ( (az + GRAV_ACC*cosd(pit) ) / velX) * RAD2DEG * DELTA_T_pullUp;

        velDOld = velD;
        if abs(pit) < gammaMax
            % third step - g on set rate with pull up G

            az = az - gRate*GRAV_ACC*DELTA_T_pullUp;
            az = saturate(az, -upGMax*GRAV_ACC, upGMax*GRAV_ACC);
            aTmp = [0, 0, az]';
%             fprintf('gRate: %.2f, az: %.2f \r\n', gRate, az);
            [accNED, ~] = convertBody2NED([rol, pit, hdg], aTmp);

            velN = velN + accNED(1)*DELTA_T_pullUp;
            velE = velE + accNED(2)*DELTA_T_pullUp;
            velD = velD + accNED(3)*DELTA_T_pullUp;

        else
            % fourth step - Maximum flight path angle rising
            pit = sign(pit) * gammaMax;
        end

        % [3.3] Update Position
        % Rate of change in geodetic coordinates [deg/s]
        velLatOld = velLat;
        velLonOld = velLon;
        velLat  = velN / latLength;
        velLon  = velE / lonLength;

        pullUpTraj(ii, 1, 1) = pullUpTraj(ii-1, 1, 1) + (velLat + velLatOld)/2 * DELTA_T;
        pullUpTraj(ii, 1, 2) = pullUpTraj(ii-1, 1, 2) + (velLon + velLonOld)/2 * DELTA_T;
        pullUpTraj(ii, 1, 3) = pullUpTraj(ii-1, 1, 3) - (velD + velDOld)/2 * DELTA_T;

    end

end

end

%% Internal functions
function [latLength, lonLength] = getLengthOfADegree(lat, h)
%GETLENGTHOFADEGREE
% Calculate the length of one degree of both latitude and longitude
% for a specified latitude and height
%
% == Inputs =========
% lat               - Latitude [deg]
% h                 - Height [m]
% 
% == Outputs ========
% latLength         - Length of 1 deg of latitude on the ref. spheroid [m]
% lonLength         - Length of 1 deg of longitude on the ref. spheroid [m]
% ===================

% WGS84 Parameters
eRadius = 6378137.0;
eEccen = 0.08181919;

% Radius of curvature in prime vertical
nE = eRadius / sqrt( 1 - (eEccen^2*(sind(lat))^2) );
% Meridian Radius of Curavature
mE = eRadius * (1 - eEccen^2) / (1 - eEccen^2*(sind(lat))^2)^(1.5);

lonLength = (nE + h) * cosd(lat) * (pi/180);
latLength = (mE + h) * (pi/180);

end

function [vecNED, C_b_n] = convertBody2NED(eulerDeg, vecXYZ)
%CONVERTBODY2NED 동체 좌표계 벡터를 NED 좌표계 벡터로 변환
% Body2NED 변환 행렬 출력

% Initialize
vecNED = zeros(3,1);
C_b_n = zeros(3,3);

% Trigonometirc functions
cRol = cosd(eulerDeg(1));
sRol = sind(eulerDeg(1));
cPit = cosd(eulerDeg(2));
sPit = sind(eulerDeg(2));
cYaw = cosd(eulerDeg(3));
sYaw = sind(eulerDeg(3));

% Transformation matrix
C_b_n   = [cPit*cYaw, sRol*sPit*cYaw-cRol*sYaw, cRol*sPit*cYaw+sRol*sYaw; ...
           cPit*sYaw, sRol*sPit*sYaw+cRol*cYaw, cRol*sPit*sYaw-sRol*cYaw; ...
               -sPit,                sRol*cPit,                cRol*cPit];

vecNED = C_b_n * vecXYZ;

end

function out = saturate(in, minVal, maxVal)
%SATURATE
% Saturates input value to [min, max]
%
% == Inputs =========
% in                - input value
% minVal            - minimum value
% maxVal            - maximum value
% == Outputs ========
% out               - saturated output value
% ===================

out = min(maxVal, max(minVal, in));

end

== matlab function GCAWS/ImplementGCAWS/HullProfile/ConfigureSWH ==
  data: newSWH input; swhUsing output; oldSWH input
function swhUsing = ConfigureSWH(newSWH, oldSWH)
%ConfigureSWH

swhUsing = single(0.0);

if ( newSWH >= 0.0 ) && ( newSWH < 1524.0 )
    swhUsing = single(newSWH);
elseif ( oldSWH >= 0.0 ) && ( oldSWH < 1524.0 )
    swhUsing = single(oldSWH);
else
    swhUsing = single(15.24);
end

end

== matlab function GCAWS/ImplementGCAWS/UpdateOutput/CheckGCAWSParameterValidity ==
  data: paramSel input; reactionTime input; valid output; rollRate input; gOnsetRate input; pullUpG input; maxFlightPathAngle input
function valid = CheckParamValid(paramSel, reactionTime, rollRate, gOnsetRate, pullUpG, maxFlightPathAngle)
%CheckParamValid

% Initialize
arrValid    = zeros(6, 1, 'logical');
valid       = false;

% Test
arrValid(1)     = paramSel;
arrValid(2)     = (reactionTime < uint16(4));
arrValid(3)     = (rollRate < uint16(4));
arrValid(4)     = (gOnsetRate < uint16(4));
arrValid(5)     = (pullUpG < uint16(4));
arrValid(6)     = (maxFlightPathAngle < uint16(4));

% Result
valid = all(arrValid);
